simulink model "step_encoder_recording"  (R2018a)
settings: Solver=FixedStepDiscrete  StartTime=0.0  StopTime=10.0  RelTol=1e-3
PreLoadFcn:
  | waijung.modelPreload; % Required for working with Waijung Blockset. Do not remove.
undefined symbols (not defined in the file or in its folder): HSEOSC, Link, LQFP144, ST, STM32F446ZE
libraries: simulink x14, stm32f4_io_lib x7, commsynccomp2 x2, stm32f4_device_config_lib x1, dspbuff3 x1, stm32f4_tim_lib x1
(part 2 of 4)

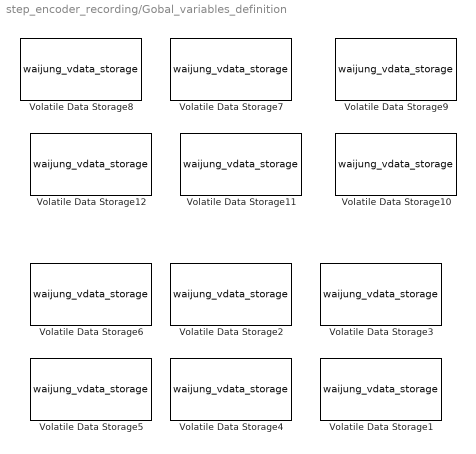
== system step_encoder_recording/Gobal_variables_definition ==
  Volatile Data Storage1 : S-Function  FunctionName=waijung_vdata_storage  Parameters=storagetype,storagename,initval,varname,buffersize,initvalstring,sampletime,sampletimestr,blockid,storagetypestr  SFunctionDeploymentMode=off  EnableBusSupport=off  mask(waijung_vdata_storage){storagetype=single, definevolatile=on, storagename=Laser, initval=90, varname=Gobal_variables_definitionVolatileDataStorage1_Laser, buffersize=64, initvalstring='Initial string', webintegration=Disable, weboutputformat='%f', webcgicallback=(void*)0, laststoragetype=single, sampletime=-1, sampletimestr=-1, blockid=Gobal_variables_definitionVolatileDataStorage1, storagetypestr=volatile float}
      mask prompts: storagetype "Storage Type"; definevolatile "Define with "volatile" keyword"; storagename "Storage Name (must be a valid variable name)"; initval "Initial value (Apply at Power on Reset only)"; varname "Variable name"; buffersize "Size (bytes)"; initvalstring "Initial value (Apply at Power on Reset only)"; webintegration "Web CGI varget/varset integration"; weboutputformat "Web CGI varget output format"; webcgicallback "Web CGI varset callback"; laststoragetype "Last selected Storage Type"; sampletime "Sample time (sec)"; sampletimestr "Compiled sample time (sec) in string"; storagetypestr "Type string"
      mask help:
      | This block implements a volatile Data Storage.
      |
      | Web CGI varset/varget integratiopn:
      | Enable - In webserver application, allow remote access via http.
      | Disable - Variable is use in local only.
      mask init:
      | waijung_vdata_storage_callback('init');
      mask Help: web(fullfile(waijungdocroot,'Volatile_Data_Storage.htm'))
      mask TypeOptions storagetype: double | single | uint32 | int32 | uint16 | int16 | uint8 | int8 | string
      mask Callback storagetype: waijung_vdata_storage_callback('storagetype');
      mask Callback storagename: waijung_vdata_storage_callback('storagename');
      mask Callback initval: waijung_vdata_storage_callback('initval');
      mask Callback varname: waijung_vdata_storage_callback('varname');
      mask Callback initvalstring: waijung_vdata_storage_callback('initvalstring');
      mask TypeOptions webintegration: Disable | ReadOnly | Write/ Read | ReadOnly with KeyValuePair | Write/ Read with KeyValuePair
      mask Callback webintegration: waijung_vdata_storage_callback('webintegration');
      mask Callback weboutputformat: waijung_vdata_storage_callback('weboutputformat');
      mask TypeOptions laststoragetype: double | single | uint32 | int32 | uint16 | int16 | uint8 | int8 | string
      mask Callback sampletime: waijung_vdata_storage_callback('sampletime');
      mask Callback sampletimestr: waijung_vdata_storage_callback('sampletimestr');
      mask Callback blockid: waijung_vdata_storage_callback('blockid');
      mask Display: text(0.5, 0.5, 'Name: Laser\nType: single','ver','middle','hor','center')
  Volatile Data Storage10 : S-Function  FunctionName=waijung_vdata_storage  Parameters=storagetype,storagename,initval,varname,buffersize,initvalstring,sampletime,sampletimestr,blockid,storagetypestr  SFunctionDeploymentMode=off  EnableBusSupport=off  mask(waijung_vdata_storage){storagetype=uint16, definevolatile=on, storagename=DDS_TUNE2, initval=3, varname=VolatileDataStorage3_DDS_TUNE, buffersize=64, initvalstring='Initial string', webintegration=Disable, weboutputformat='%u', webcgicallback=(void*)0, laststoragetype=uint16, sampletime=-1, sampletimestr=-1, blockid=Gobal_variables_definitionVolatileDataStorage10, storagetypestr=volatile uint16_t}
      mask prompts: storagetype "Storage Type"; definevolatile "Define with "volatile" keyword"; storagename "Storage Name (must be a valid variable name)"; initval "Initial value (Apply at Power on Reset only)"; varname "Variable name"; buffersize "Size (bytes)"; initvalstring "Initial value (Apply at Power on Reset only)"; webintegration "Web CGI varget/varset integration"; weboutputformat "Web CGI varget output format"; webcgicallback "Web CGI varset callback"; laststoragetype "Last selected Storage Type"; sampletime "Sample time (sec)"; sampletimestr "Compiled sample time (sec) in string"; storagetypestr "Type string"
      mask help:
      | This block implements a volatile Data Storage.
      |
      | Web CGI varset/varget integratiopn:
      | Enable - In webserver application, allow remote access via http.
      | Disable - Variable is use in local only.
      mask init:
      | waijung_vdata_storage_callback('init');
      mask Help: web(fullfile(waijungdocroot,'Volatile_Data_Storage.htm'))
      mask TypeOptions storagetype: double | single | uint32 | int32 | uint16 | int16 | uint8 | int8 | string
      mask Callback storagetype: waijung_vdata_storage_callback('storagetype');
      mask Callback storagename: waijung_vdata_storage_callback('storagename');
      mask Callback initval: waijung_vdata_storage_callback('initval');
      mask Callback varname: waijung_vdata_storage_callback('varname');
      mask Callback initvalstring: waijung_vdata_storage_callback('initvalstring');
      mask TypeOptions webintegration: Disable | ReadOnly | Write/ Read | ReadOnly with KeyValuePair | Write/ Read with KeyValuePair
      mask Callback webintegration: waijung_vdata_storage_callback('webintegration');
      mask Callback weboutputformat: waijung_vdata_storage_callback('weboutputformat');
      mask TypeOptions laststoragetype: double | single | uint32 | int32 | uint16 | int16 | uint8 | int8 | string
      mask Callback sampletime: waijung_vdata_storage_callback('sampletime');
      mask Callback sampletimestr: waijung_vdata_storage_callback('sampletimestr');
      mask Callback blockid: waijung_vdata_storage_callback('blockid');
      mask Display: text(0.5, 0.5, 'Name: DDS_TUNE2\nType: uint16','ver','middle','hor','center')
  Volatile Data Storage11 : S-Function  FunctionName=waijung_vdata_storage  Parameters=storagetype,storagename,initval,varname,buffersize,initvalstring,sampletime,sampletimestr,blockid,storagetypestr  SFunctionDeploymentMode=off  EnableBusSupport=off  mask(waijung_vdata_storage){storagetype=uint16, definevolatile=on, storagename=DDS_ACC2, initval=0, varname=VolatileDataStorage1_DDS_ACC, buffersize=64, initvalstring='Initial string', webintegration=Disable, weboutputformat='%u', webcgicallback=(void*)0, laststoragetype=uint16, sampletime=-1, sampletimestr=-1, blockid=Gobal_variables_definitionVolatileDataStorage11, storagetypestr=volatile uint16_t}
      mask prompts: storagetype "Storage Type"; definevolatile "Define with "volatile" keyword"; storagename "Storage Name (must be a valid variable name)"; initval "Initial value (Apply at Power on Reset only)"; varname "Variable name"; buffersize "Size (bytes)"; initvalstring "Initial value (Apply at Power on Reset only)"; webintegration "Web CGI varget/varset integration"; weboutputformat "Web CGI varget output format"; webcgicallback "Web CGI varset callback"; laststoragetype "Last selected Storage Type"; sampletime "Sample time (sec)"; sampletimestr "Compiled sample time (sec) in string"; storagetypestr "Type string"
      mask help:
      | This block implements a volatile Data Storage.
      |
      | Web CGI varset/varget integratiopn:
      | Enable - In webserver application, allow remote access via http.
      | Disable - Variable is use in local only.
      mask init:
      | waijung_vdata_storage_callback('init');
      mask Help: web(fullfile(waijungdocroot,'Volatile_Data_Storage.htm'))
      mask TypeOptions storagetype: double | single | uint32 | int32 | uint16 | int16 | uint8 | int8 | string
      mask Callback storagetype: waijung_vdata_storage_callback('storagetype');
      mask Callback storagename: waijung_vdata_storage_callback('storagename');
      mask Callback initval: waijung_vdata_storage_callback('initval');
      mask Callback varname: waijung_vdata_storage_callback('varname');
      mask Callback initvalstring: waijung_vdata_storage_callback('initvalstring');
      mask TypeOptions webintegration: Disable | ReadOnly | Write/ Read | ReadOnly with KeyValuePair | Write/ Read with KeyValuePair
      mask Callback webintegration: waijung_vdata_storage_callback('webintegration');
      mask Callback weboutputformat: waijung_vdata_storage_callback('weboutputformat');
      mask TypeOptions laststoragetype: double | single | uint32 | int32 | uint16 | int16 | uint8 | int8 | string
      mask Callback sampletime: waijung_vdata_storage_callback('sampletime');
      mask Callback sampletimestr: waijung_vdata_storage_callback('sampletimestr');
      mask Callback blockid: waijung_vdata_storage_callback('blockid');
      mask Display: text(0.5, 0.5, 'Name: DDS_ACC2\nType: uint16','ver','middle','hor','center')
  Volatile Data Storage12 : S-Function  FunctionName=waijung_vdata_storage  Parameters=storagetype,storagename,initval,varname,buffersize,initvalstring,sampletime,sampletimestr,blockid,storagetypestr  SFunctionDeploymentMode=off  EnableBusSupport=off  mask(waijung_vdata_storage){storagetype=uint16, definevolatile=on, storagename=DDS_MASK2, initval=hex2dec('1000'), varname=VolatileDataStorage2_DDS_MASK, buffersize=64, initvalstring='Initial string', webintegration=Disable, weboutputformat='%u', webcgicallback=(void*)0, laststoragetype=uint16, sampletime=-1, sampletimestr=-1, blockid=Gobal_variables_definitionVolatileDataStorage12, storagetypestr=volatile uint16_t}
      mask prompts: storagetype "Storage Type"; definevolatile "Define with "volatile" keyword"; storagename "Storage Name (must be a valid variable name)"; initval "Initial value (Apply at Power on Reset only)"; varname "Variable name"; buffersize "Size (bytes)"; initvalstring "Initial value (Apply at Power on Reset only)"; webintegration "Web CGI varget/varset integration"; weboutputformat "Web CGI varget output format"; webcgicallback "Web CGI varset callback"; laststoragetype "Last selected Storage Type"; sampletime "Sample time (sec)"; sampletimestr "Compiled sample time (sec) in string"; storagetypestr "Type string"
      mask help:
      | This block implements a volatile Data Storage.
      |
      | Web CGI varset/varget integratiopn:
      | Enable - In webserver application, allow remote access via http.
      | Disable - Variable is use in local only.
      mask init:
      | waijung_vdata_storage_callback('init');
      mask Help: web(fullfile(waijungdocroot,'Volatile_Data_Storage.htm'))
      mask TypeOptions storagetype: double | single | uint32 | int32 | uint16 | int16 | uint8 | int8 | string
      mask Callback storagetype: waijung_vdata_storage_callback('storagetype');
      mask Callback storagename: waijung_vdata_storage_callback('storagename');
      mask Callback initval: waijung_vdata_storage_callback('initval');
      mask Callback varname: waijung_vdata_storage_callback('varname');
      mask Callback initvalstring: waijung_vdata_storage_callback('initvalstring');
      mask TypeOptions webintegration: Disable | ReadOnly | Write/ Read | ReadOnly with KeyValuePair | Write/ Read with KeyValuePair
      mask Callback webintegration: waijung_vdata_storage_callback('webintegration');
      mask Callback weboutputformat: waijung_vdata_storage_callback('weboutputformat');
      mask TypeOptions laststoragetype: double | single | uint32 | int32 | uint16 | int16 | uint8 | int8 | string
      mask Callback sampletime: waijung_vdata_storage_callback('sampletime');
      mask Callback sampletimestr: waijung_vdata_storage_callback('sampletimestr');
      mask Callback blockid: waijung_vdata_storage_callback('blockid');
      mask Display: text(0.5, 0.5, 'Name: DDS_MASK2\nType: uint16','ver','middle','hor','center')
  Volatile Data Storage2 : S-Function  FunctionName=waijung_vdata_storage  Parameters=storagetype,storagename,initval,varname,buffersize,initvalstring,sampletime,sampletimestr,blockid,storagetypestr  SFunctionDeploymentMode=off  EnableBusSupport=off  mask(waijung_vdata_storage){storagetype=double, definevolatile=on, storagename=Ax, initval=0, varname=Gobal_variables_definitionVolatileDataStorage2_Ax, buffersize=64, initvalstring='Initial string', webintegration=Disable, weboutputformat='%f', webcgicallback=(void*)0, laststoragetype=double, sampletime=-1, sampletimestr=-1, blockid=Gobal_variables_definitionVolatileDataStorage2, storagetypestr=volatile double}
      mask prompts: storagetype "Storage Type"; definevolatile "Define with "volatile" keyword"; storagename "Storage Name (must be a valid variable name)"; initval "Initial value (Apply at Power on Reset only)"; varname "Variable name"; buffersize "Size (bytes)"; initvalstring "Initial value (Apply at Power on Reset only)"; webintegration "Web CGI varget/varset integration"; weboutputformat "Web CGI varget output format"; webcgicallback "Web CGI varset callback"; laststoragetype "Last selected Storage Type"; sampletime "Sample time (sec)"; sampletimestr "Compiled sample time (sec) in string"; storagetypestr "Type string"
      mask help:
      | This block implements a volatile Data Storage.
      |
      | Web CGI varset/varget integratiopn:
      | Enable - In webserver application, allow remote access via http.
      | Disable - Variable is use in local only.
      mask init:
      | waijung_vdata_storage_callback('init');
      mask Help: web(fullfile(waijungdocroot,'Volatile_Data_Storage.htm'))
      mask TypeOptions storagetype: double | single | uint32 | int32 | uint16 | int16 | uint8 | int8 | string
      mask Callback storagetype: waijung_vdata_storage_callback('storagetype');
      mask Callback storagename: waijung_vdata_storage_callback('storagename');
      mask Callback initval: waijung_vdata_storage_callback('initval');
      mask Callback varname: waijung_vdata_storage_callback('varname');
      mask Callback initvalstring: waijung_vdata_storage_callback('initvalstring');
      mask TypeOptions webintegration: Disable | ReadOnly | Write/ Read | ReadOnly with KeyValuePair | Write/ Read with KeyValuePair
      mask Callback webintegration: waijung_vdata_storage_callback('webintegration');
      mask Callback weboutputformat: waijung_vdata_storage_callback('weboutputformat');
      mask TypeOptions laststoragetype: double | single | uint32 | int32 | uint16 | int16 | uint8 | int8 | string
      mask Callback sampletime: waijung_vdata_storage_callback('sampletime');
      mask Callback sampletimestr: waijung_vdata_storage_callback('sampletimestr');
      mask Callback blockid: waijung_vdata_storage_callback('blockid');
      mask Display: text(0.5, 0.5, 'Name: Ax\nType: double','ver','middle','hor','center')
  Volatile Data Storage3 : S-Function  FunctionName=waijung_vdata_storage  Parameters=storagetype,storagename,initval,varname,buffersize,initvalstring,sampletime,sampletimestr,blockid,storagetypestr  SFunctionDeploymentMode=off  EnableBusSupport=off  mask(waijung_vdata_storage){storagetype=uint8, definevolatile=on, storagename=flag, initval=0, varname=Gobal_variables_definitionVolatileDataStorage3_flag, buffersize=64, initvalstring='Initial string', webintegration=Disable, weboutputformat='%u', webcgicallback=(void*)0, laststoragetype=uint8, sampletime=-1, sampletimestr=-1, blockid=Gobal_variables_definitionVolatileDataStorage3, storagetypestr=volatile uint8_t}
      mask prompts: storagetype "Storage Type"; definevolatile "Define with "volatile" keyword"; storagename "Storage Name (must be a valid variable name)"; initval "Initial value (Apply at Power on Reset only)"; varname "Variable name"; buffersize "Size (bytes)"; initvalstring "Initial value (Apply at Power on Reset only)"; webintegration "Web CGI varget/varset integration"; weboutputformat "Web CGI varget output format"; webcgicallback "Web CGI varset callback"; laststoragetype "Last selected Storage Type"; sampletime "Sample time (sec)"; sampletimestr "Compiled sample time (sec) in string"; storagetypestr "Type string"
      mask help:
      | This block implements a volatile Data Storage.
      |
      | Web CGI varset/varget integratiopn:
      | Enable - In webserver application, allow remote access via http.
      | Disable - Variable is use in local only.
      mask init:
      | waijung_vdata_storage_callback('init');
      mask Help: web(fullfile(waijungdocroot,'Volatile_Data_Storage.htm'))
      mask TypeOptions storagetype: double | single | uint32 | int32 | uint16 | int16 | uint8 | int8 | string
      mask Callback storagetype: waijung_vdata_storage_callback('storagetype');
      mask Callback storagename: waijung_vdata_storage_callback('storagename');
      mask Callback initval: waijung_vdata_storage_callback('initval');
      mask Callback varname: waijung_vdata_storage_callback('varname');
      mask Callback initvalstring: waijung_vdata_storage_callback('initvalstring');
      mask TypeOptions webintegration: Disable | ReadOnly | Write/ Read | ReadOnly with KeyValuePair | Write/ Read with KeyValuePair
      mask Callback webintegration: waijung_vdata_storage_callback('webintegration');
      mask Callback weboutputformat: waijung_vdata_storage_callback('weboutputformat');
      mask TypeOptions laststoragetype: double | single | uint32 | int32 | uint16 | int16 | uint8 | int8 | string
      mask Callback sampletime: waijung_vdata_storage_callback('sampletime');
      mask Callback sampletimestr: waijung_vdata_storage_callback('sampletimestr');
      mask Callback blockid: waijung_vdata_storage_callback('blockid');
      mask Display: text(0.5, 0.5, 'Name: flag\nType: uint8','ver','middle','hor','center')
  Volatile Data Storage4 : S-Function  FunctionName=waijung_vdata_storage  Parameters=storagetype,storagename,initval,varname,buffersize,initvalstring,sampletime,sampletimestr,blockid,storagetypestr  SFunctionDeploymentMode=off  EnableBusSupport=off  mask(waijung_vdata_storage){storagetype=double, definevolatile=on, storagename=fx, initval=0, varname=Gobal_variables_definitionVolatileDataStorage4_fx, buffersize=64, initvalstring='Initial string', webintegration=Disable, weboutputformat='%f', webcgicallback=(void*)0, laststoragetype=double, sampletime=-1, sampletimestr=-1, blockid=Gobal_variables_definitionVolatileDataStorage4, storagetypestr=volatile double}
      mask prompts: storagetype "Storage Type"; definevolatile "Define with "volatile" keyword"; storagename "Storage Name (must be a valid variable name)"; initval "Initial value (Apply at Power on Reset only)"; varname "Variable name"; buffersize "Size (bytes)"; initvalstring "Initial value (Apply at Power on Reset only)"; webintegration "Web CGI varget/varset integration"; weboutputformat "Web CGI varget output format"; webcgicallback "Web CGI varset callback"; laststoragetype "Last selected Storage Type"; sampletime "Sample time (sec)"; sampletimestr "Compiled sample time (sec) in string"; storagetypestr "Type string"
      mask help:
      | This block implements a volatile Data Storage.
      |
      | Web CGI varset/varget integratiopn:
      | Enable - In webserver application, allow remote access via http.
      | Disable - Variable is use in local only.
      mask init:
      | waijung_vdata_storage_callback('init');
      mask Help: web(fullfile(waijungdocroot,'Volatile_Data_Storage.htm'))
      mask TypeOptions storagetype: double | single | uint32 | int32 | uint16 | int16 | uint8 | int8 | string
      mask Callback storagetype: waijung_vdata_storage_callback('storagetype');
      mask Callback storagename: waijung_vdata_storage_callback('storagename');
      mask Callback initval: waijung_vdata_storage_callback('initval');
      mask Callback varname: waijung_vdata_storage_callback('varname');
      mask Callback initvalstring: waijung_vdata_storage_callback('initvalstring');
      mask TypeOptions webintegration: Disable | ReadOnly | Write/ Read | ReadOnly with KeyValuePair | Write/ Read with KeyValuePair
      mask Callback webintegration: waijung_vdata_storage_callback('webintegration');
      mask Callback weboutputformat: waijung_vdata_storage_callback('weboutputformat');
      mask TypeOptions laststoragetype: double | single | uint32 | int32 | uint16 | int16 | uint8 | int8 | string
      mask Callback sampletime: waijung_vdata_storage_callback('sampletime');
      mask Callback sampletimestr: waijung_vdata_storage_callback('sampletimestr');
      mask Callback blockid: waijung_vdata_storage_callback('blockid');
      mask Display: text(0.5, 0.5, 'Name: fx\nType: double','ver','middle','hor','center')
  Volatile Data Storage5 : S-Function  FunctionName=waijung_vdata_storage  Parameters=storagetype,storagename,initval,varname,buffersize,initvalstring,sampletime,sampletimestr,blockid,storagetypestr  SFunctionDeploymentMode=off  EnableBusSupport=off  mask(waijung_vdata_storage){storagetype=double, definevolatile=on, storagename=fy, initval=0, varname=Gobal_variables_definitionVolatileDataStorage5_fy, buffersize=64, initvalstring='Initial string', webintegration=Disable, weboutputformat='%f', webcgicallback=(void*)0, laststoragetype=double, sampletime=-1, sampletimestr=-1, blockid=Gobal_variables_definitionVolatileDataStorage5, storagetypestr=volatile double}
      mask prompts: storagetype "Storage Type"; definevolatile "Define with "volatile" keyword"; storagename "Storage Name (must be a valid variable name)"; initval "Initial value (Apply at Power on Reset only)"; varname "Variable name"; buffersize "Size (bytes)"; initvalstring "Initial value (Apply at Power on Reset only)"; webintegration "Web CGI varget/varset integration"; weboutputformat "Web CGI varget output format"; webcgicallback "Web CGI varset callback"; laststoragetype "Last selected Storage Type"; sampletime "Sample time (sec)"; sampletimestr "Compiled sample time (sec) in string"; storagetypestr "Type string"
      mask help:
      | This block implements a volatile Data Storage.
      |
      | Web CGI varset/varget integratiopn:
      | Enable - In webserver application, allow remote access via http.
      | Disable - Variable is use in local only.
      mask init:
      | waijung_vdata_storage_callback('init');
      mask Help: web(fullfile(waijungdocroot,'Volatile_Data_Storage.htm'))
      mask TypeOptions storagetype: double | single | uint32 | int32 | uint16 | int16 | uint8 | int8 | string
      mask Callback storagetype: waijung_vdata_storage_callback('storagetype');
      mask Callback storagename: waijung_vdata_storage_callback('storagename');
      mask Callback initval: waijung_vdata_storage_callback('initval');
      mask Callback varname: waijung_vdata_storage_callback('varname');
      mask Callback initvalstring: waijung_vdata_storage_callback('initvalstring');
      mask TypeOptions webintegration: Disable | ReadOnly | Write/ Read | ReadOnly with KeyValuePair | Write/ Read with KeyValuePair
      mask Callback webintegration: waijung_vdata_storage_callback('webintegration');
      mask Callback weboutputformat: waijung_vdata_storage_callback('weboutputformat');
      mask TypeOptions laststoragetype: double | single | uint32 | int32 | uint16 | int16 | uint8 | int8 | string
      mask Callback sampletime: waijung_vdata_storage_callback('sampletime');
      mask Callback sampletimestr: waijung_vdata_storage_callback('sampletimestr');
      mask Callback blockid: waijung_vdata_storage_callback('blockid');
      mask Display: text(0.5, 0.5, 'Name: fy\nType: double','ver','middle','hor','center')
  Volatile Data Storage6 : S-Function  FunctionName=waijung_vdata_storage  Parameters=storagetype,storagename,initval,varname,buffersize,initvalstring,sampletime,sampletimestr,blockid,storagetypestr  SFunctionDeploymentMode=off  EnableBusSupport=off  mask(waijung_vdata_storage){storagetype=double, definevolatile=on, storagename=Ay, initval=0, varname=Gobal_variables_definitionVolatileDataStorage6_Ay, buffersize=64, initvalstring='Initial string', webintegration=Disable, weboutputformat='%f', webcgicallback=(void*)0, laststoragetype=double, sampletime=-1, sampletimestr=-1, blockid=Gobal_variables_definitionVolatileDataStorage6, storagetypestr=volatile double}
      mask prompts: storagetype "Storage Type"; definevolatile "Define with "volatile" keyword"; storagename "Storage Name (must be a valid variable name)"; initval "Initial value (Apply at Power on Reset only)"; varname "Variable name"; buffersize "Size (bytes)"; initvalstring "Initial value (Apply at Power on Reset only)"; webintegration "Web CGI varget/varset integration"; weboutputformat "Web CGI varget output format"; webcgicallback "Web CGI varset callback"; laststoragetype "Last selected Storage Type"; sampletime "Sample time (sec)"; sampletimestr "Compiled sample time (sec) in string"; storagetypestr "Type string"
      mask help:
      | This block implements a volatile Data Storage.
      |
      | Web CGI varset/varget integratiopn:
      | Enable - In webserver application, allow remote access via http.
      | Disable - Variable is use in local only.
      mask init:
      | waijung_vdata_storage_callback('init');
      mask Help: web(fullfile(waijungdocroot,'Volatile_Data_Storage.htm'))
      mask TypeOptions storagetype: double | single | uint32 | int32 | uint16 | int16 | uint8 | int8 | string
      mask Callback storagetype: waijung_vdata_storage_callback('storagetype');
      mask Callback storagename: waijung_vdata_storage_callback('storagename');
      mask Callback initval: waijung_vdata_storage_callback('initval');
      mask Callback varname: waijung_vdata_storage_callback('varname');
      mask Callback initvalstring: waijung_vdata_storage_callback('initvalstring');
      mask TypeOptions webintegration: Disable | ReadOnly | Write/ Read | ReadOnly with KeyValuePair | Write/ Read with KeyValuePair
      mask Callback webintegration: waijung_vdata_storage_callback('webintegration');
      mask Callback weboutputformat: waijung_vdata_storage_callback('weboutputformat');
      mask TypeOptions laststoragetype: double | single | uint32 | int32 | uint16 | int16 | uint8 | int8 | string
      mask Callback sampletime: waijung_vdata_storage_callback('sampletime');
      mask Callback sampletimestr: waijung_vdata_storage_callback('sampletimestr');
      mask Callback blockid: waijung_vdata_storage_callback('blockid');
      mask Display: text(0.5, 0.5, 'Name: Ay\nType: double','ver','middle','hor','center')
  Volatile Data Storage7 : S-Function  FunctionName=waijung_vdata_storage  Parameters=storagetype,storagename,initval,varname,buffersize,initvalstring,sampletime,sampletimestr,blockid,storagetypestr  SFunctionDeploymentMode=off  EnableBusSupport=off  mask(waijung_vdata_storage){storagetype=uint16, definevolatile=on, storagename=DDS_ACC1, initval=0, varname=VolatileDataStorage1_DDS_ACC, buffersize=64, initvalstring='Initial string', webintegration=Disable, weboutputformat='%u', webcgicallback=(void*)0, laststoragetype=uint16, sampletime=-1, sampletimestr=-1, blockid=Gobal_variables_definitionVolatileDataStorage7, storagetypestr=volatile uint16_t}
      mask prompts: storagetype "Storage Type"; definevolatile "Define with "volatile" keyword"; storagename "Storage Name (must be a valid variable name)"; initval "Initial value (Apply at Power on Reset only)"; varname "Variable name"; buffersize "Size (bytes)"; initvalstring "Initial value (Apply at Power on Reset only)"; webintegration "Web CGI varget/varset integration"; weboutputformat "Web CGI varget output format"; webcgicallback "Web CGI varset callback"; laststoragetype "Last selected Storage Type"; sampletime "Sample time (sec)"; sampletimestr "Compiled sample time (sec) in string"; storagetypestr "Type string"
      mask help:
      | This block implements a volatile Data Storage.
      |
      | Web CGI varset/varget integratiopn:
      | Enable - In webserver application, allow remote access via http.
      | Disable - Variable is use in local only.
      mask init:
      | waijung_vdata_storage_callback('init');
      mask Help: web(fullfile(waijungdocroot,'Volatile_Data_Storage.htm'))
      mask TypeOptions storagetype: double | single | uint32 | int32 | uint16 | int16 | uint8 | int8 | string
      mask Callback storagetype: waijung_vdata_storage_callback('storagetype');
      mask Callback storagename: waijung_vdata_storage_callback('storagename');
      mask Callback initval: waijung_vdata_storage_callback('initval');
      mask Callback varname: waijung_vdata_storage_callback('varname');
      mask Callback initvalstring: waijung_vdata_storage_callback('initvalstring');
      mask TypeOptions webintegration: Disable | ReadOnly | Write/ Read | ReadOnly with KeyValuePair | Write/ Read with KeyValuePair
      mask Callback webintegration: waijung_vdata_storage_callback('webintegration');
      mask Callback weboutputformat: waijung_vdata_storage_callback('weboutputformat');
      mask TypeOptions laststoragetype: double | single | uint32 | int32 | uint16 | int16 | uint8 | int8 | string
      mask Callback sampletime: waijung_vdata_storage_callback('sampletime');
      mask Callback sampletimestr: waijung_vdata_storage_callback('sampletimestr');
      mask Callback blockid: waijung_vdata_storage_callback('blockid');
      mask Display: text(0.5, 0.5, 'Name: DDS_ACC1\nType: uint16','ver','middle','hor','center')
  Volatile Data Storage8 : S-Function  FunctionName=waijung_vdata_storage  Parameters=storagetype,storagename,initval,varname,buffersize,initvalstring,sampletime,sampletimestr,blockid,storagetypestr  SFunctionDeploymentMode=off  EnableBusSupport=off  mask(waijung_vdata_storage){storagetype=uint16, definevolatile=on, storagename=DDS_MASK1, initval=hex2dec('1000'), varname=VolatileDataStorage2_DDS_MASK, buffersize=64, initvalstring='Initial string', webintegration=Disable, weboutputformat='%u', webcgicallback=(void*)0, laststoragetype=uint16, sampletime=-1, sampletimestr=-1, blockid=Gobal_variables_definitionVolatileDataStorage8, storagetypestr=volatile uint16_t}
      mask prompts: storagetype "Storage Type"; definevolatile "Define with "volatile" keyword"; storagename "Storage Name (must be a valid variable name)"; initval "Initial value (Apply at Power on Reset only)"; varname "Variable name"; buffersize "Size (bytes)"; initvalstring "Initial value (Apply at Power on Reset only)"; webintegration "Web CGI varget/varset integration"; weboutputformat "Web CGI varget output format"; webcgicallback "Web CGI varset callback"; laststoragetype "Last selected Storage Type"; sampletime "Sample time (sec)"; sampletimestr "Compiled sample time (sec) in string"; storagetypestr "Type string"
      mask help:
      | This block implements a volatile Data Storage.
      |
      | Web CGI varset/varget integratiopn:
      | Enable - In webserver application, allow remote access via http.
      | Disable - Variable is use in local only.
      mask init:
      | waijung_vdata_storage_callback('init');
      mask Help: web(fullfile(waijungdocroot,'Volatile_Data_Storage.htm'))
      mask TypeOptions storagetype: double | single | uint32 | int32 | uint16 | int16 | uint8 | int8 | string
      mask Callback storagetype: waijung_vdata_storage_callback('storagetype');
      mask Callback storagename: waijung_vdata_storage_callback('storagename');
      mask Callback initval: waijung_vdata_storage_callback('initval');
      mask Callback varname: waijung_vdata_storage_callback('varname');
      mask Callback initvalstring: waijung_vdata_storage_callback('initvalstring');
      mask TypeOptions webintegration: Disable | ReadOnly | Write/ Read | ReadOnly with KeyValuePair | Write/ Read with KeyValuePair
      mask Callback webintegration: waijung_vdata_storage_callback('webintegration');
      mask Callback weboutputformat: waijung_vdata_storage_callback('weboutputformat');
      mask TypeOptions laststoragetype: double | single | uint32 | int32 | uint16 | int16 | uint8 | int8 | string
      mask Callback sampletime: waijung_vdata_storage_callback('sampletime');
      mask Callback sampletimestr: waijung_vdata_storage_callback('sampletimestr');
      mask Callback blockid: waijung_vdata_storage_callback('blockid');
      mask Display: text(0.5, 0.5, 'Name: DDS_MASK1\nType: uint16','ver','middle','hor','center')
  Volatile Data Storage9 : S-Function  FunctionName=waijung_vdata_storage  Parameters=storagetype,storagename,initval,varname,buffersize,initvalstring,sampletime,sampletimestr,blockid,storagetypestr  SFunctionDeploymentMode=off  EnableBusSupport=off  mask(waijung_vdata_storage){storagetype=uint16, definevolatile=on, storagename=DDS_TUNE1, initval=3, varname=VolatileDataStorage3_DDS_TUNE, buffersize=64, initvalstring='Initial string', webintegration=Disable, weboutputformat='%u', webcgicallback=(void*)0, laststoragetype=uint16, sampletime=-1, sampletimestr=-1, blockid=Gobal_variables_definitionVolatileDataStorage9, storagetypestr=volatile uint16_t}
      mask prompts: storagetype "Storage Type"; definevolatile "Define with "volatile" keyword"; storagename "Storage Name (must be a valid variable name)"; initval "Initial value (Apply at Power on Reset only)"; varname "Variable name"; buffersize "Size (bytes)"; initvalstring "Initial value (Apply at Power on Reset only)"; webintegration "Web CGI varget/varset integration"; weboutputformat "Web CGI varget output format"; webcgicallback "Web CGI varset callback"; laststoragetype "Last selected Storage Type"; sampletime "Sample time (sec)"; sampletimestr "Compiled sample time (sec) in string"; storagetypestr "Type string"
      mask help:
      | This block implements a volatile Data Storage.
      |
      | Web CGI varset/varget integratiopn:
      | Enable - In webserver application, allow remote access via http.
      | Disable - Variable is use in local only.
      mask init:
      | waijung_vdata_storage_callback('init');
      mask Help: web(fullfile(waijungdocroot,'Volatile_Data_Storage.htm'))
      mask TypeOptions storagetype: double | single | uint32 | int32 | uint16 | int16 | uint8 | int8 | string
      mask Callback storagetype: waijung_vdata_storage_callback('storagetype');
      mask Callback storagename: waijung_vdata_storage_callback('storagename');
      mask Callback initval: waijung_vdata_storage_callback('initval');
      mask Callback varname: waijung_vdata_storage_callback('varname');
      mask Callback initvalstring: waijung_vdata_storage_callback('initvalstring');
      mask TypeOptions webintegration: Disable | ReadOnly | Write/ Read | ReadOnly with KeyValuePair | Write/ Read with KeyValuePair
      mask Callback webintegration: waijung_vdata_storage_callback('webintegration');
      mask Callback weboutputformat: waijung_vdata_storage_callback('weboutputformat');
      mask TypeOptions laststoragetype: double | single | uint32 | int32 | uint16 | int16 | uint8 | int8 | string
      mask Callback sampletime: waijung_vdata_storage_callback('sampletime');
      mask Callback sampletimestr: waijung_vdata_storage_callback('sampletimestr');
      mask Callback blockid: waijung_vdata_storage_callback('blockid');
      mask Display: text(0.5, 0.5, 'Name: DDS_TUNE1\nType: uint16','ver','middle','hor','center')

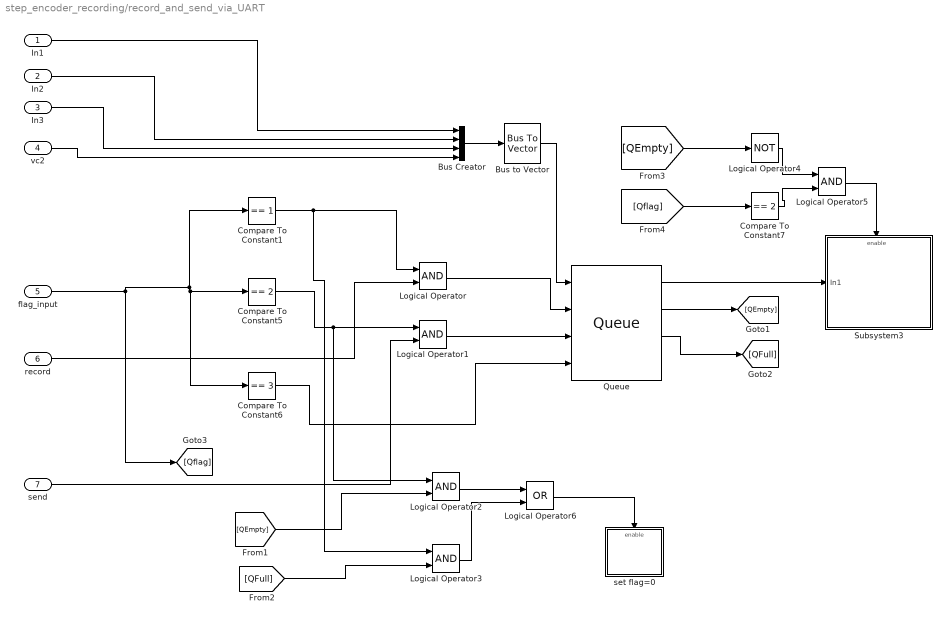
== system step_encoder_recording/record_and_send_via_UART ==
  In1 : Inport
  In2 : Inport  Port=2
  In3 : Inport  Port=3
  vc2 : Inport  Port=4
  flag_input : Inport  Port=5
  record : Inport  Port=6
  send : Inport  Port=7
  Bus Creator : BusCreator  Inputs=4
  Bus to Vector : BusToVector
  Compare To Constant1 : simulink/Logic and Bit Operations/Compare To Constant  relop===  const=1  OutDataTypeStr=boolean
  Compare To Constant5 : simulink/Logic and Bit Operations/Compare To Constant  relop===  const=2  OutDataTypeStr=boolean
  Compare To Constant6 : simulink/Logic and Bit Operations/Compare To Constant  relop===  const=3  OutDataTypeStr=boolean
  Compare To Constant7 : simulink/Logic and Bit Operations/Compare To Constant  relop===  const=2  OutDataTypeStr=boolean
  Logical Operator{,1..3,5} (5 alike) : Logic  AllPortsSameDT=off  OutDataTypeStr=boolean
  Logical Operator4 : Logic  Operator=NOT  AllPortsSameDT=off  OutDataTypeStr=boolean
  Logical Operator6 : Logic  Operator=OR  AllPortsSameDT=off  OutDataTypeStr=boolean
  Queue : dspbuff3/Queue  depth=3000  trigger=Either edge  overflow=Ignore  pes=Ignore  eso=on  fso=on  nso=on  clr=on  clrOutport=on  adf=on
      settings: SourceProductName=DSP System Toolbox  SourceProductBaseCode=DS
  Subsystem3 : Subsystem
  set flag=0 : Subsystem
  wires:
  send/1 -> Logical Operator1/2
  [QFull] -> Logical Operator3/2
  Logical Operator/1 -> Queue/2
  record/1 -> Logical Operator/2
  Logical Operator1/1 -> Queue/3
  Queue/2 -> [QEmpty]
  Logical Operator3/1 -> Logical Operator6/2
  Compare To Constant7/1 -> Logical Operator5/2
  Compare To Constant5/1 -> Logical Operator1/1, Logical Operator2/1
  Compare To Constant1/1 -> Logical Operator3/1, Logical Operator/1
  [QEmpty] -> Logical Operator2/2
  Compare To Constant6/1 -> Queue/4
  [QEmpty] -> Logical Operator4/1
  Logical Operator4/1 -> Logical Operator5/1
  Queue/3 -> [QFull]
  [Qflag] -> Compare To Constant7/1
  Logical Operator5/1 -> Subsystem3/Enable
  Logical Operator6/1 -> set flag=0/Enable
  Bus Creator/1 -> Bus to Vector/1
  Bus to Vector/1 -> Queue/1
  In2/1 -> Bus Creator/2
  Logical Operator2/1 -> Logical Operator6/1
  In1/1 -> Bus Creator/1
  Queue/1 -> Subsystem3/1(In1)
  flag_input/1 -> Compare To Constant6/1, Compare To Constant5/1, Compare To Constant1/1, [Qflag]
  In3/1 -> Bus Creator/3
  vc2/1 -> Bus Creator/4
